simulink model "observe_2021a"  (R2021a)
settings: Solver=FixedStepAuto  StartTime=0.0  StopTime=15  RelTol=1e-3
model workspace (MAT data in the model file):
  A = 1
values from neighbouring files (symbols this model uses):
  Ap = [0, 1, 0; -C*df0*I0/mass, 0, -2*C*f0*I0/mass; 0, 0, -R/L]    [sliding_mode_control.m]    (also in system_state_feedback.m = [0, 1, 0; -C*df0*I0^2/mass, 0, -2*C*f0*I0/mass; 0, 0, -R/L]; system_state_feedback_observer.m = [0, 1, 0; -C*df0*I0^2/mass, 0, -2*C*f0*I0/mass; 0, 0, -R/L])
  Bp = [0; 0; 1/L]    [sliding_mode_control.m]    (also in system_state_feedback.m; system_state_feedback_observer.m)
  Cp = [1, 0, 0; 1, 0, 1]    [sliding_mode_control.m]    (also in system_state_feedback.m = [1, 0, 0; 0, 0, 1]; system_state_feedback_observer.m = [1, 0, 0; 0, 0, 1])
  D = [-C*df0*I0^2/mass-lambda^2, -2*C*f0*I0/mass]    [system_state_feedback_observer.m]
  I0 = sqrt((mass*grav)/(C*f_mag_y(y0)))    [sliding_mode_control.m]    (also in system_state_feedback.m = f_I0(y0); system_state_feedback_observer.m)
  K = place(Ap,Bp,p)    [sliding_mode_control.m]    (also in system_state_feedback.m; system_state_feedback_observer.m)
  L = 3.165    [feedback_linealization.m]    (also in sliding_mode_control.m; system_state_feedback.m; system_state_feedback_observer.m = place(Apt,Cpt,q))
  lambda = 200    [system_state_feedback_observer.m]
  V = [1,0;lambda,0;0,1]    [system_state_feedback_observer.m]
  V0 = R*I0    [sliding_mode_control.m]    (also in system_state_feedback.m = f_V0(y0); system_state_feedback_observer.m)
  W = [0;1;0]    [system_state_feedback_observer.m]
  y0 = 0.018    [sliding_mode_control.m]    (also in system_state_feedback.m = 0.03; system_state_feedback_observer.m = 0.02)
undefined symbols (not defined in the file or in its folder): National_Instruments, PCIe
libraries: sldrtlib x7
settings Model: SimulationMode=external  Creator=磁気浮上  LastModifiedBy=磁気浮上
settings SolverCC: AlgebraicLoopSolver=TrustRegion  DecoupledContinuousIntegration=on  MinimalZcImpactIntegration=on
settings DataIOCC: ReturnWorkspaceOutputs=off
settings DebuggingCC: SFMachineParentedDataDiag=warning  ArithmeticOperatorsInVariantConditions=warning
settings SFSimCC: SimUseLocalCustomCode=off  CustomCodeUndefinedFunction=UseInterfaceOnly
settings RTWCC: Description=Simulink Desktop Real-Time  SystemTargetFile=sldrt.tlc  TemplateMakefile=sldrt.tmf  RTWUseLocalCustomCode=off  RTWCompilerOptimization=on
settings CodeAppCC: MaxIdLength=95
settings SimulinkDesktopRealTimeCC: TargetPreCompLibLocation=C:\Program Files\MATLAB\R2021a\toolbox\sldrt\lib\win64

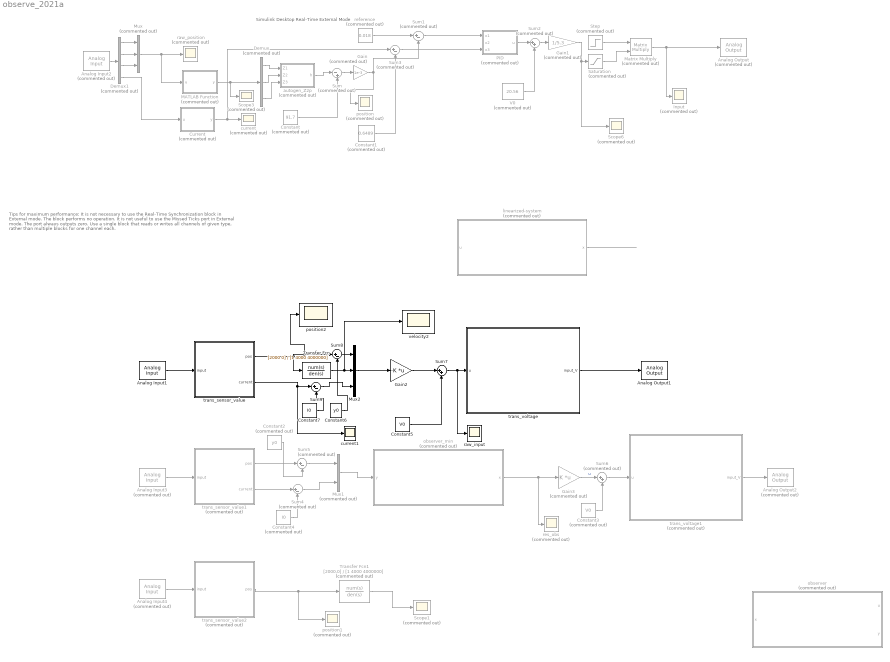
== system observe_2021a ==
  note: Simulink Desktop Real-Time External Mode
  note: Tips for maximum performance:
      |
      | It is not necessary to use the Real-Time Synchronization block in External mode. The block performs no operation.
      | It is not useful to use the Missed Ticks port in External mode. The port always outputs zero.
      | Use a single block that reads or writes all channels of given type, rather than multiple blocks for one channel each.
  Analog Input1 : sldrtlib/Analog Input  SampleTime=0.001  MaxMissedTicks=10  ShowMissedTicks=off  YieldWhenWaiting=off  DrvName=National_Instruments/PCIe-6361  DrvAddress=4294967295  DrvOptions=[0 0 0 0 0 0 0]  Channels=[1 2 3 5]  RangeMode=1  VoltRange=1  DataType=1
      settings: AttributesFormatString=National Instruments\nPCIe-6361 [auto]
  Analog Input2 : sldrtlib/Analog Input  Commented=on  SampleTime=0.001  MaxMissedTicks=10  ShowMissedTicks=off  YieldWhenWaiting=off  DrvName=National_Instruments/PCIe-6361  DrvAddress=4294967295  DrvOptions=[0 0 0 0 0 0 0]  Channels=[1 2 3 5]  RangeMode=1  VoltRange=1  DataType=1
      settings: AttributesFormatString=National Instruments\nPCIe-6361 [auto]
  Analog Input3 : sldrtlib/Analog Input  Commented=on  SampleTime=0.001  MaxMissedTicks=10  ShowMissedTicks=off  YieldWhenWaiting=off  DrvName=National_Instruments/PCIe-6361  DrvAddress=4294967295  DrvOptions=[0 0 0 0 0 0 0]  Channels=[1 2 3 5]  RangeMode=1  VoltRange=1  DataType=1
      settings: AttributesFormatString=National Instruments\nPCIe-6361 [auto]
  Analog Input4 : sldrtlib/Analog Input  Commented=on  SampleTime=0.0005  MaxMissedTicks=10  ShowMissedTicks=off  YieldWhenWaiting=off  DrvName=National_Instruments/PCIe-6361  DrvAddress=4294967295  DrvOptions=[0 0 0 0 0 0 0]  Channels=[1 2 3]  RangeMode=1  VoltRange=1  DataType=1
      settings: AttributesFormatString=National Instruments\nPCIe-6361 [auto]
  Analog Output : sldrtlib/Analog Output  Commented=on  SampleTime=0.001  MaxMissedTicks=10  ShowMissedTicks=off  YieldWhenWaiting=off  DrvName=National_Instruments/PCIe-6361  DrvAddress=4294967295  DrvOptions=[0 0 0 0 0 0 0]  Channels=1  RangeMode=1  VoltRange=1  InitialValue=[]  FinalValue=[]
      settings: AttributesFormatString=National Instruments\nPCIe-6361 [auto]
  Analog Output1 : sldrtlib/Analog Output  SampleTime=0.001  MaxMissedTicks=10  ShowMissedTicks=off  YieldWhenWaiting=off  DrvName=National_Instruments/PCIe-6361  DrvAddress=4294967295  DrvOptions=[0 0 0 0 0 0 0]  Channels=1  RangeMode=1  VoltRange=1  InitialValue=[]  FinalValue=[]
      settings: AttributesFormatString=National Instruments\nPCIe-6361 [auto]
  Analog Output2 : sldrtlib/Analog Output  Commented=on  SampleTime=0.001  MaxMissedTicks=10  ShowMissedTicks=off  YieldWhenWaiting=off  DrvName=National_Instruments/PCIe-6361  DrvAddress=4294967295  DrvOptions=[0 0 0 0 0 0 0]  Channels=1  RangeMode=1  VoltRange=1  InitialValue=[]  FinalValue=[]
      settings: AttributesFormatString=National Instruments\nPCIe-6361 [auto]
  Constant : Constant  Commented=on  Value=91.7
  Constant1 : Constant  Commented=on  Value=0.6489
  Constant2 : Constant  Commented=on  Value=y0
  Constant3 : Constant  Commented=on  Value=V0
  Constant4 : Constant  Commented=on  Value=I0
  Constant5 : Constant  Value=V0
  Constant6 : Constant  Value=y0
  Constant7 : Constant  Value=I0
  Current : MATLAB Function  Commented=on  TreatAsAtomicUnit=on
  Demux : Demux  Commented=on  Outputs=3
  Demux1 : Demux  Commented=on
  Gain : Gain  Commented=on  Gain=1e-3
  Gain1 : Gain  Commented=on  Gain=1/5.3
  Gain2 : Gain  Gain=-K  Multiplication=Matrix(K*u)
  Gain3 : Gain  Commented=on  Gain=K  Multiplication=Matrix(K*u)
  Input : Scope  Commented=on
  MATLAB Function : MATLAB Function  Commented=on  TreatAsAtomicUnit=on
  Matrix Multiply : Product  Commented=on  Multiplication=Matrix(*)
  Mux : Mux  Commented=on  Inputs=3
  Mux1 : Mux  Commented=on  Inputs=2
  Mux2 : Mux  Inputs=3
  PID : MATLAB Function  Commented=on  TreatAsAtomicUnit=on
  Saturation : Saturate  Commented=on  UpperLimit=10  LowerLimit=-10
  Scope1 : Scope  Commented=on
  Scope3 : Scope  Commented=on
  Scope6 : Scope  Commented=on
  Step : Step  Commented=on  Time=15  Before=1  After=0  SampleTime=0
  Sum : Sum  Commented=on  Inputs=|-+
  Sum{1,3..5} (4 alike) : Sum  Commented=on  Inputs=|+-
  Sum2 : Sum  Commented=on  Inputs=|++
  Sum6 : Sum  Commented=on  Inputs=|++
  Sum7 : Sum  Inputs=|++
  Sum8 : Sum  Inputs=|+-
  Sum9 : Sum  Inputs=|+-
  Transfer Fcn : TransferFcn  Numerator=[2000 0]  Denominator=[1 4000 4000000]
  Transfer Fcn1 : TransferFcn  Commented=on  Numerator=[2000,0]  Denominator=[1 4000 4000000]
  V0 : Constant  Commented=on  Value=20.56
  autogen_Z2p : MATLAB Function  Commented=on  TreatAsAtomicUnit=on
  current : Scope  Commented=on
  current1 : Scope
  linearized-system : Subsystem  Commented=on
  observer : Subsystem  Commented=on
  observer_min : Subsystem  Commented=on
  position : Scope  Commented=on
  position1 : Scope  Commented=on
  position2 : Scope
  raw_input : Scope
  raw_position : Scope  Commented=on
  reference : Constant  Commented=on  Value=0.018
  res_obs : Scope  Commented=on
  trans_sensor_value : Subsystem
  trans_sensor_value1 : Subsystem  Commented=on
  trans_sensor_value2 : Subsystem  Commented=on
  trans_voltage : Subsystem
  trans_voltage1 : Subsystem  Commented=on
  velocity2 : Scope
  wires:
  Step/1 -> Matrix Multiply/1
  Constant/1 -> Sum/2
  autogen_Z2p/1(h) -> Sum/1
  Matrix Multiply/1 -> Analog Output/1, Input/1
  MATLAB Function/1(y) -> Scope3/1, Demux/1
  Sum/1 -> Gain/1
  Demux/2 -> autogen_Z2p/2(Z2)
  Demux/1 -> autogen_Z2p/1(Z1)
  Saturation/1 -> Matrix Multiply/2
  Demux/3 -> autogen_Z2p/3(Z3)
  Current/1(y) -> Sum3/1, current/1
  Analog Input2/1 -> Demux1/1
  Demux1/1 -> Mux/1
  Demux1/4 -> Current/1(u)
  Demux1/3 -> Mux/3
  Demux1/2 -> Mux/2
  Mux/1 -> MATLAB Function/1(u), raw_position/1
  Gain/1 -> Sum1/2, position/1
  reference/1 -> Sum1/1
  Sum1/1 -> PID/1(x1)
  V0/1 -> Sum2/2
  PID/1(u) -> Sum2/1
  Sum2/1 -> Gain1/1
  Gain1/1 -> Saturation/1, Scope6/1
  Sum3/1 -> PID/3(x3)
  Constant1/1 -> Sum3/2
  linearized-system/1(x) -> ?
  Analog Input1/1 -> trans_sensor_value/1(input)
  trans_sensor_value/1(pos) -> position2/1, Sum8/1, Transfer Fcn/1
  trans_sensor_value/2(current) -> Sum9/1, current1/1
  Gain2/1 -> Sum7/1
  trans_voltage/1(input_V) -> Analog Output1/1
  trans_voltage1/1(input_V) -> Analog Output2/1
  trans_sensor_value1/1(pos) -> Sum5/1
  Analog Input3/1 -> trans_sensor_value1/1(input)
  Gain3/1 -> Sum6/1  "u"
  Transfer Fcn/1 -> velocity2/1, Mux2/2
  Mux2/1 -> Gain2/1
  Mux1/1 -> observer_min/1(y)
  observer_min/1(x) -> res_obs/1, Gain3/1
  Constant4/1 -> Sum4/2
  trans_sensor_value1/2(current) -> Sum4/1
  Sum4/1 -> Mux1/2
  Constant2/1 -> Sum5/2
  Sum5/1 -> Mux1/1
  Constant3/1 -> Sum6/2
  Sum6/1 -> trans_voltage1/1(u)
  trans_sensor_value2/1(pos) -> position1/1, Transfer Fcn1/1
  Transfer Fcn1/1 -> Scope1/1
  Analog Input4/1 -> trans_sensor_value2/1(input)
  Constant5/1 -> Sum7/2
  Sum7/1 -> raw_input/1, trans_voltage/1(u)
  Constant6/1 -> Sum8/2
  Sum8/1 -> Mux2/1
  Constant7/1 -> Sum9/2
  Sum9/1 -> Mux2/3

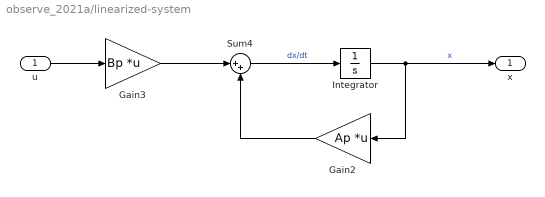
== system observe_2021a/linearized-system ==
  u : Inport
  Gain2 : Gain  Gain=Ap  Multiplication=Matrix(K*u)
  Gain3 : Gain  Gain=Bp  Multiplication=Matrix(K*u)
  Integrator : Integrator
  Sum4 : Sum  Inputs=|++
  x : Outport
  wires:
  Gain3/1 -> Sum4/1
  Gain2/1 -> Sum4/2
  u/1 -> Gain3/1
  Integrator/1 -> Gain2/1, x/1  "x"
  Sum4/1 -> Integrator/1  "dx/dt"

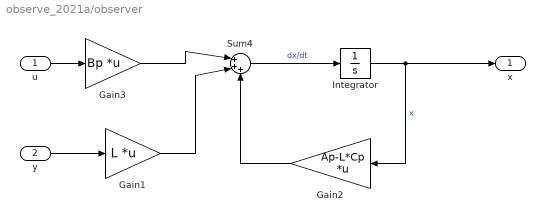
== system observe_2021a/observer ==
  u : Inport
  y : Inport  Port=2
  Gain1 : Gain  Gain=L  Multiplication=Matrix(K*u)
  Gain2 : Gain  Gain=Ap-L*Cp  Multiplication=Matrix(K*u)
  Gain3 : Gain  Gain=Bp  Multiplication=Matrix(K*u)
  Integrator : Integrator
  Sum4 : Sum  Inputs=|+++
  x : Outport
  wires:
  Gain3/1 -> Sum4/1
  Gain2/1 -> Sum4/3
  Integrator/1 -> Gain2/1, x/1  "x"
  Sum4/1 -> Integrator/1  "dx/dt"
  y/1 -> Gain1/1
  Gain1/1 -> Sum4/2
  u/1 -> Gain3/1

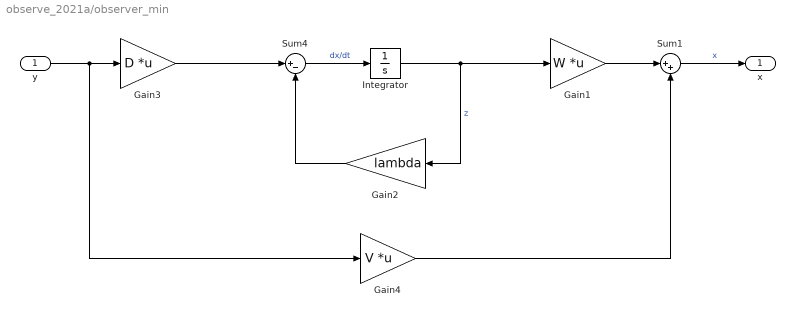
== system observe_2021a/observer_min ==
  y : Inport
  Gain1 : Gain  Gain=W  Multiplication=Matrix(K*u)
  Gain2 : Gain  Gain=lambda
  Gain3 : Gain  Gain=D  Multiplication=Matrix(K*u)
  Gain4 : Gain  Gain=V  Multiplication=Matrix(K*u)
  Integrator : Integrator
  Sum1 : Sum  Inputs=|++
  Sum4 : Sum  Inputs=|+-
  x : Outport
  wires:
  Gain2/1 -> Sum4/2
  Integrator/1 -> Gain1/1, Gain2/1  "z"
  Sum4/1 -> Integrator/1  "dx/dt"
  y/1 -> Gain4/1, Gain3/1
  Gain3/1 -> Sum4/1
  Gain1/1 -> Sum1/1
  Gain4/1 -> Sum1/2
  Sum1/1 -> x/1  "x"

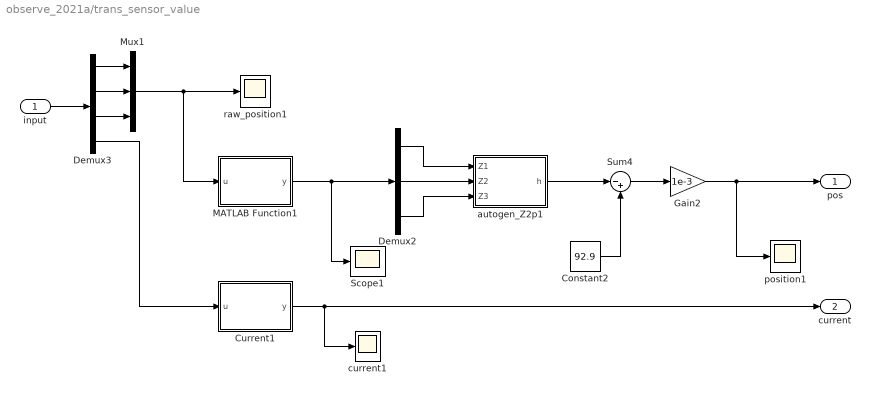
== system observe_2021a/trans_sensor_value ==
  input : Inport
  Constant2 : Constant  Value=92.9
  Current1 : MATLAB Function  TreatAsAtomicUnit=on
  Demux2 : Demux  Outputs=3
  Demux3 : Demux
  Gain2 : Gain  Gain=1e-3
  MATLAB Function1 : MATLAB Function  TreatAsAtomicUnit=on
  Mux1 : Mux  Inputs=3
  Scope1 : Scope
  Sum4 : Sum  Inputs=|-+
  autogen_Z2p1 : MATLAB Function  TreatAsAtomicUnit=on
  current1 : Scope
  position1 : Scope
  raw_position1 : Scope
  pos : Outport
  current : Outport  Port=2
  wires:
  Gain2/1 -> pos/1, position1/1
  MATLAB Function1/1(y) -> Demux2/1, Scope1/1
  Mux1/1 -> MATLAB Function1/1(u), raw_position1/1
  Sum4/1 -> Gain2/1
  Demux3/1 -> Mux1/1
  Demux2/1 -> autogen_Z2p1/1(Z1)
  autogen_Z2p1/1(h) -> Sum4/1
  Demux3/3 -> Mux1/3
  Demux2/3 -> autogen_Z2p1/3(Z3)
  Demux2/2 -> autogen_Z2p1/2(Z2)
  Demux3/4 -> Current1/1(u)
  Demux3/2 -> Mux1/2
  Current1/1(y) -> current/1, current1/1
  Constant2/1 -> Sum4/2
  input/1 -> Demux3/1

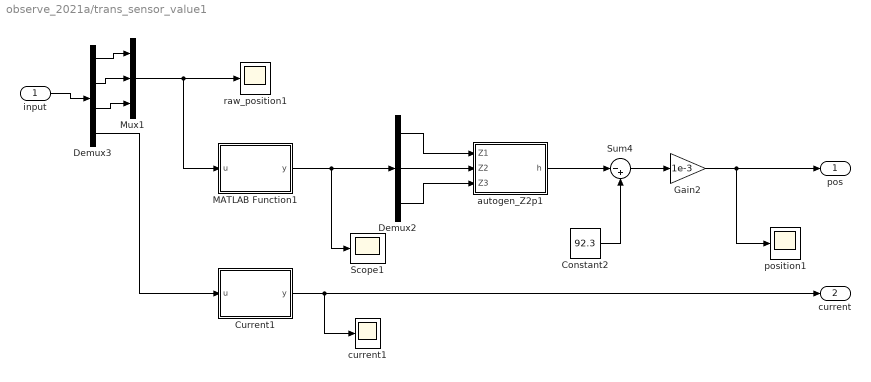
== system observe_2021a/trans_sensor_value1 ==
  input : Inport
  Constant2 : Constant  Value=92.3
  Current1 : MATLAB Function  TreatAsAtomicUnit=on
  Demux2 : Demux  Outputs=3
  Demux3 : Demux
  Gain2 : Gain  Gain=1e-3
  MATLAB Function1 : MATLAB Function  TreatAsAtomicUnit=on
  Mux1 : Mux  Inputs=3
  Scope1 : Scope
  Sum4 : Sum  Inputs=|-+
  autogen_Z2p1 : MATLAB Function  TreatAsAtomicUnit=on
  current1 : Scope
  position1 : Scope
  raw_position1 : Scope
  pos : Outport
  current : Outport  Port=2
  wires:
  Gain2/1 -> pos/1, position1/1
  MATLAB Function1/1(y) -> Demux2/1, Scope1/1
  Mux1/1 -> MATLAB Function1/1(u), raw_position1/1
  Sum4/1 -> Gain2/1
  Demux3/1 -> Mux1/1
  Demux2/1 -> autogen_Z2p1/1(Z1)
  autogen_Z2p1/1(h) -> Sum4/1
  Demux3/3 -> Mux1/3
  Demux2/3 -> autogen_Z2p1/3(Z3)
  Demux2/2 -> autogen_Z2p1/2(Z2)
  Demux3/4 -> Current1/1(u)
  Demux3/2 -> Mux1/2
  Current1/1(y) -> current/1, current1/1
  Constant2/1 -> Sum4/2
  input/1 -> Demux3/1

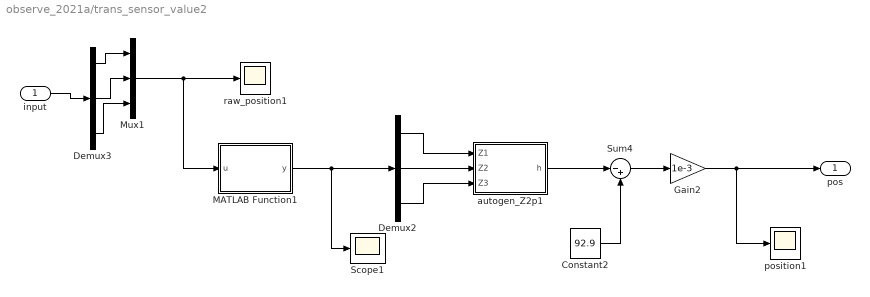
== system observe_2021a/trans_sensor_value2 ==
  input : Inport
  Constant2 : Constant  Value=92.9
  Demux2 : Demux  Outputs=3
  Demux3 : Demux  Outputs=3
  Gain2 : Gain  Gain=1e-3
  MATLAB Function1 : MATLAB Function  TreatAsAtomicUnit=on
  Mux1 : Mux  Inputs=3
  Scope1 : Scope
  Sum4 : Sum  Inputs=|-+
  autogen_Z2p1 : MATLAB Function  TreatAsAtomicUnit=on
  position1 : Scope
  raw_position1 : Scope
  pos : Outport
  wires:
  Gain2/1 -> pos/1, position1/1
  MATLAB Function1/1(y) -> Demux2/1, Scope1/1
  Mux1/1 -> MATLAB Function1/1(u), raw_position1/1
  Sum4/1 -> Gain2/1
  Demux3/1 -> Mux1/1
  Demux2/1 -> autogen_Z2p1/1(Z1)
  autogen_Z2p1/1(h) -> Sum4/1
  Demux3/3 -> Mux1/3
  Demux2/3 -> autogen_Z2p1/3(Z3)
  Demux2/2 -> autogen_Z2p1/2(Z2)
  Demux3/2 -> Mux1/2
  Constant2/1 -> Sum4/2
  input/1 -> Demux3/1

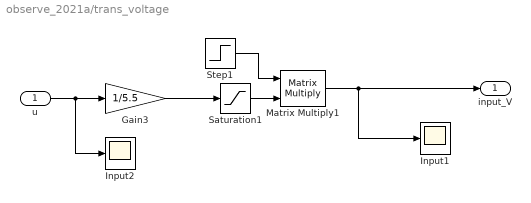
== system observe_2021a/trans_voltage ==
  u : Inport
  Gain3 : Gain  Gain=1/5.5
  Input1 : Scope
  Input2 : Scope
  Matrix Multiply1 : Product  Multiplication=Matrix(*)
  Saturation1 : Saturate  UpperLimit=10  LowerLimit=-10
  Step1 : Step  Time=10  Before=1  After=0  SampleTime=0
  input_V : Outport
  wires:
  Gain3/1 -> Saturation1/1
  Step1/1 -> Matrix Multiply1/1
  Matrix Multiply1/1 -> input_V/1, Input1/1
  u/1 -> Input2/1, Gain3/1
  Saturation1/1 -> Matrix Multiply1/2

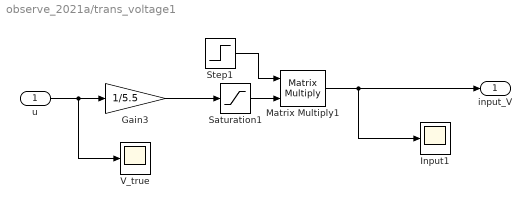
== system observe_2021a/trans_voltage1 ==
  u : Inport
  Gain3 : Gain  Gain=1/5.5
  Input1 : Scope
  Matrix Multiply1 : Product  Multiplication=Matrix(*)
  Saturation1 : Saturate  UpperLimit=10  LowerLimit=-10
  Step1 : Step  Time=15  Before=1  After=0  SampleTime=0
  V_true : Scope
  input_V : Outport
  wires:
  Gain3/1 -> Saturation1/1
  Step1/1 -> Matrix Multiply1/1
  Matrix Multiply1/1 -> input_V/1, Input1/1
  Saturation1/1 -> Matrix Multiply1/2
  u/1 -> V_true/1, Gain3/1

== matlab function observe_2021a/autogen_Z2p ==
  data: Z1 input; h output; Z2 input; Z3 input
function h = autogen_Z2p(Z1,Z2,Z3)
%#codegen

%    This function was generated by the Symbolic Math Toolbox version 8.7.
%    09-Feb-2022 18:15:15

t2 = Z1.^2;
t3 = Z1.^3;
t4 = Z2.^2;
t5 = Z2.^3;
t6 = Z3.^2;
t7 = Z3.^3;
t8 = Z1.*3.21e+2;
t9 = Z2.*1.297e+3;
t10 = Z3.*1.763e+3;
t11 = Z3.*2.576e+3;
t12 = Z2.*2.897e+3;
t13 = Z1.*3.06e+3;
t24 = Z2.*Z3.*1.0352122e+11;
t25 = Z2.*Z3.*2.0704244e+11;
t26 = Z1.*Z3.*9.135768e+10;
t27 = Z1.*Z3.*1.8271536e+11;
t28 = Z1.*Z2.*1.9595028e+11;
t29 = Z1.*Z2.*9.797514e+10;
t39 = Z1.*4.8999911281101e+13;
t41 = Z3.*4.7733218776365e+13;
t48 = Z2.*4.6020599945112e+13;
t56 = Z1.*Z3.*2.511664935e+13;
t57 = Z1.*1.42753730002578e+14;
t58 = Z2.*Z3.*5.124007469e+13;
t68 = Z1.*Z2.*4.264372839e+13;
t80 = Z1.*Z2.*1.7692425141e+14;
t82 = Z1.*Z3.*1.4293441815e+14;
t88 = Z2.*Z3.*2.2089361633e+14;
t14 = -t12;
t15 = -t13;
t16 = t2.*3.21e+6;
t17 = t4.*1.297e+7;
t18 = t6.*1.763e+7;
t19 = t6.*2.576e+7;
t20 = t4.*2.897e+7;
t21 = t2.*3.06e+7;
t30 = t4.*2.0149636e+11;
t31 = Z1.*t6.*4.567884e+10;
t32 = Z3.*t2.*4.567884e+10;
t33 = t2.*9.466641e+10;
t34 = t3.*9.466641e+10;
t35 = -t24;
t36 = t2.*1.8933282e+11;
t37 = -t25;
t38 = -t26;
t40 = t6.*1.948789e+11;
t42 = Z2.*t6.*5.176061e+10;
t43 = Z3.*t4.*5.176061e+10;
t44 = t4.*1.0074818e+11;
t45 = t5.*1.0074818e+11;
t46 = -t27;
t47 = -t28;
t49 = t6.*9.743945e+10;
t50 = t7.*9.743945e+10;
t51 = Z1.*t4.*4.898757e+10;
t52 = Z2.*t2.*4.898757e+10;
t53 = -t29;
t54 = Z2.*t3.*3.21e+10;
t55 = Z3.*t3.*3.21e+10;
t59 = Z1.*t7.*2.576e+11;
t60 = Z2.*t7.*2.576e+11;
t61 = Z1.*t7.*1.763e+11;
t62 = Z2.*t7.*1.763e+11;
t63 = Z1.*t5.*1.297e+11;
t64 = Z3.*t5.*1.297e+11;
t65 = Z2.*Z3.*t2.*4.66e+10;
t66 = Z2.*t3.*3.06e+11;
t67 = Z3.*t3.*3.06e+11;
t69 = Z1.*t5.*2.897e+11;
t70 = Z3.*t5.*2.897e+11;
t72 = t2.*1.699491663e+13;
t73 = Z1.*Z3.*t4.*4.823e+11;
t74 = Z2.*Z3.*t2.*5.473e+11;
t75 = Z1.*Z2.*t6.*4.357e+11;
t76 = Z1.*Z3.*t4.*2.255e+11;
t77 = -t58;
t79 = t2.*3.388018887e+13;
t84 = t4.*t6.*4.66e+10;
t86 = t6.*4.584717173e+13;
t87 = Z1.*Z2.*t6.*3.218e+11;
t91 = t4.*8.912494397e+13;
t92 = t2.*t6.*4.823e+11;
t93 = t4.*t6.*5.473e+11;
t94 = t2.*t4.*4.357e+11;
t96 = t2.*t6.*2.255e+11;
t98 = -t80;
t99 = t6.*9.788848349e+13;
t103 = t2.*t4.*3.218e+11;
t104 = -t88;
t105 = t4.*1.1408216305e+14;
t110 = t2.*2.85507460005156e+18;
t22 = -t20;
t23 = -t21;
t71 = -t55;
t78 = -t60;
t81 = -t62;
t83 = -t63;
t85 = -t66;
t89 = -t70;
t90 = -t73;
t95 = -t76;
t97 = -t79;
t100 = t8+t11+t14;
t101 = -t86;
t102 = -t87;
t106 = -t92;
t107 = -t96;
t108 = t9+t10+t15;
t109 = -t103;
t117 = t30+t36+t37+t40+t46+t47+1.42753730002578e+14;
t118 = t33+t35+t38+t44+t49+t53+7.1376865001289e+13;
t111 = t16+t19+t22-2.275477497e+9;
t112 = t17+t18+t23+3.0399800799e+10;
t119 = 1.0./t118;
t120 = 1.0./t117;
t113 = t111.^2;
t114 = t112.^2;
t115 = t100.*t111;
t116 = t108.*t112;
t121 = t110+t113+t114-2.569567140046404e+21;
t122 = t57+t115+t116;
t123 = t122.^2;
t125 = t118.*t121;
t124 = t123.*1.0e+4;
t126 = -t125;
t127 = t124+t126;
t128 = sqrt(t127);
t129 = t128./1.0e+2;
t130 = Z1.*t128.*3.799498679230342e-3;
t131 = Z1.*t128.*3.621952011976588e-2;
t132 = Z2.*t128.*1.535186849520796e-2;
t133 = Z3.*t128.*2.086765162455792e-2;
t134 = Z3.*t128.*3.049068098971141e-2;
t135 = Z2.*t128.*3.429017966894175e-2;
mt1 = [(t119.*(t61+t64+t65+t67+t72+t75+t77+t81+t82+t83+t84+t85+t90+t94+t98+t101+t105+t106+t130+t134-t135+1.922433295028705e+16))./2.0e+2,(t119.*(t61+t64+t65+t67+t72+t75+t77+t81+t82+t83+t84+t85+t90+t94+t98+t101+t105+t106-t130-t134+t135+1.922433295028705e+16))./2.0e+2,(t119.*(t54-t55+t56+t59-t60+t68+t69+t74+t89+t91+t93+t95+t97+t99+t102+t104+t107+t109+t131-t132-t133+3.556391874974202e+16))./2.0e+2];
mt2 = [(t119.*(t54+t56+t59+t68+t69+t71+t74+t78+t89+t91+t93+t95+t97+t99+t102+t104+t107+t109-t131+t132+t133+3.556391874974202e+16))./2.0e+2,t120.*(-t31-t32+t34+t39+t41-t42-t43+t45+t48+t50-t51-t52+t129)+3.0e+1,-t120.*(t31+t32-t34-t39-t41+t42+t43-t45-t48-t50+t51+t52+t129)+3.0e+1];
pv = reshape([mt1,mt2],2,3);

if pv(1,3)>0
    h=pv(1,3);
else
    h=pv(2,3);
end

== matlab function observe_2021a/trans_sensor_value/Current1 ==
  data: u input; y output
function y = fcn(u)
%u:バイポーラ電源の出力値（V）（電流を観測）、y:バイポーラ電源が流している電流(A)
    %出力電圧値が距離に変換されます。
    y=(3.01/6.23)*u;

== matlab function observe_2021a/Current ==
  data: u input; y output
function y = fcn(u)
%u:バイポーラ電源の出力値（V）（電流を観測）、y:バイポーラ電源が流している電流(A)
    %出力電圧値が距離に変換されます。
    y=(3.01/6.23)*u;

== matlab function observe_2021a/PID ==
  data: x1 input; u output; x2 input; x3 input
function u = autogen_Z2p(x1,x2,x3)
%#codegen

%    This function was generated by the Symbolic Math Toolbox version 8.7.
%    18-Apr-2022 15:37:02



K = [ -1545, -133, 6.3];
x = [x1; x2; x3];

u = -K*x;

== matlab function observe_2021a/trans_sensor_value/MATLAB Function1 ==
  data: u input; y output
function y = fcn(u)
%u:光学センサの出力(V)、y:光学センサの出力PV値(mm)
    %出力スケーリングを行っています(フリーレンジ)。（光学センサの設定10,P.4-27）
    %PV値範囲を0～-50、出力電圧範囲を-5～5としているので、以下の式に従って
    %電圧値が距離に変換されます。
    y=(u-5*ones(3,1))*(-5);
% y = u;

== matlab function observe_2021a/trans_sensor_value/autogen_Z2p1 ==
  data: Z1 input; h output; Z2 input; Z3 input
function h = autogen_Z2p(Z1,Z2,Z3)
%#codegen

%    This function was generated by the Symbolic Math Toolbox version 8.7.
%    09-Feb-2022 18:15:15

t2 = Z1.^2;
t3 = Z1.^3;
t4 = Z2.^2;
t5 = Z2.^3;
t6 = Z3.^2;
t7 = Z3.^3;
t8 = Z1.*3.21e+2;
t9 = Z2.*1.297e+3;
t10 = Z3.*1.763e+3;
t11 = Z3.*2.576e+3;
t12 = Z2.*2.897e+3;
t13 = Z1.*3.06e+3;
t24 = Z2.*Z3.*1.0352122e+11;
t25 = Z2.*Z3.*2.0704244e+11;
t26 = Z1.*Z3.*9.135768e+10;
t27 = Z1.*Z3.*1.8271536e+11;
t28 = Z1.*Z2.*1.9595028e+11;
t29 = Z1.*Z2.*9.797514e+10;
t39 = Z1.*4.8999911281101e+13;
t41 = Z3.*4.7733218776365e+13;
t48 = Z2.*4.6020599945112e+13;
t56 = Z1.*Z3.*2.511664935e+13;
t57 = Z1.*1.42753730002578e+14;
t58 = Z2.*Z3.*5.124007469e+13;
t68 = Z1.*Z2.*4.264372839e+13;
t80 = Z1.*Z2.*1.7692425141e+14;
t82 = Z1.*Z3.*1.4293441815e+14;
t88 = Z2.*Z3.*2.2089361633e+14;
t14 = -t12;
t15 = -t13;
t16 = t2.*3.21e+6;
t17 = t4.*1.297e+7;
t18 = t6.*1.763e+7;
t19 = t6.*2.576e+7;
t20 = t4.*2.897e+7;
t21 = t2.*3.06e+7;
t30 = t4.*2.0149636e+11;
t31 = Z1.*t6.*4.567884e+10;
t32 = Z3.*t2.*4.567884e+10;
t33 = t2.*9.466641e+10;
t34 = t3.*9.466641e+10;
t35 = -t24;
t36 = t2.*1.8933282e+11;
t37 = -t25;
t38 = -t26;
t40 = t6.*1.948789e+11;
t42 = Z2.*t6.*5.176061e+10;
t43 = Z3.*t4.*5.176061e+10;
t44 = t4.*1.0074818e+11;
t45 = t5.*1.0074818e+11;
t46 = -t27;
t47 = -t28;
t49 = t6.*9.743945e+10;
t50 = t7.*9.743945e+10;
t51 = Z1.*t4.*4.898757e+10;
t52 = Z2.*t2.*4.898757e+10;
t53 = -t29;
t54 = Z2.*t3.*3.21e+10;
t55 = Z3.*t3.*3.21e+10;
t59 = Z1.*t7.*2.576e+11;
t60 = Z2.*t7.*2.576e+11;
t61 = Z1.*t7.*1.763e+11;
t62 = Z2.*t7.*1.763e+11;
t63 = Z1.*t5.*1.297e+11;
t64 = Z3.*t5.*1.297e+11;
t65 = Z2.*Z3.*t2.*4.66e+10;
t66 = Z2.*t3.*3.06e+11;
t67 = Z3.*t3.*3.06e+11;
t69 = Z1.*t5.*2.897e+11;
t70 = Z3.*t5.*2.897e+11;
t72 = t2.*1.699491663e+13;
t73 = Z1.*Z3.*t4.*4.823e+11;
t74 = Z2.*Z3.*t2.*5.473e+11;
t75 = Z1.*Z2.*t6.*4.357e+11;
t76 = Z1.*Z3.*t4.*2.255e+11;
t77 = -t58;
t79 = t2.*3.388018887e+13;
t84 = t4.*t6.*4.66e+10;
t86 = t6.*4.584717173e+13;
t87 = Z1.*Z2.*t6.*3.218e+11;
t91 = t4.*8.912494397e+13;
t92 = t2.*t6.*4.823e+11;
t93 = t4.*t6.*5.473e+11;
t94 = t2.*t4.*4.357e+11;
t96 = t2.*t6.*2.255e+11;
t98 = -t80;
t99 = t6.*9.788848349e+13;
t103 = t2.*t4.*3.218e+11;
t104 = -t88;
t105 = t4.*1.1408216305e+14;
t110 = t2.*2.85507460005156e+18;
t22 = -t20;
t23 = -t21;
t71 = -t55;
t78 = -t60;
t81 = -t62;
t83 = -t63;
t85 = -t66;
t89 = -t70;
t90 = -t73;
t95 = -t76;
t97 = -t79;
t100 = t8+t11+t14;
t101 = -t86;
t102 = -t87;
t106 = -t92;
t107 = -t96;
t108 = t9+t10+t15;
t109 = -t103;
t117 = t30+t36+t37+t40+t46+t47+1.42753730002578e+14;
t118 = t33+t35+t38+t44+t49+t53+7.1376865001289e+13;
t111 = t16+t19+t22-2.275477497e+9;
t112 = t17+t18+t23+3.0399800799e+10;
t119 = 1.0./t118;
t120 = 1.0./t117;
t113 = t111.^2;
t114 = t112.^2;
t115 = t100.*t111;
t116 = t108.*t112;
t121 = t110+t113+t114-2.569567140046404e+21;
t122 = t57+t115+t116;
t123 = t122.^2;
t125 = t118.*t121;
t124 = t123.*1.0e+4;
t126 = -t125;
t127 = t124+t126;
t128 = sqrt(t127);
t129 = t128./1.0e+2;
t130 = Z1.*t128.*3.799498679230342e-3;
t131 = Z1.*t128.*3.621952011976588e-2;
t132 = Z2.*t128.*1.535186849520796e-2;
t133 = Z3.*t128.*2.086765162455792e-2;
t134 = Z3.*t128.*3.049068098971141e-2;
t135 = Z2.*t128.*3.429017966894175e-2;
mt1 = [(t119.*(t61+t64+t65+t67+t72+t75+t77+t81+t82+t83+t84+t85+t90+t94+t98+t101+t105+t106+t130+t134-t135+1.922433295028705e+16))./2.0e+2,(t119.*(t61+t64+t65+t67+t72+t75+t77+t81+t82+t83+t84+t85+t90+t94+t98+t101+t105+t106-t130-t134+t135+1.922433295028705e+16))./2.0e+2,(t119.*(t54-t55+t56+t59-t60+t68+t69+t74+t89+t91+t93+t95+t97+t99+t102+t104+t107+t109+t131-t132-t133+3.556391874974202e+16))./2.0e+2];
mt2 = [(t119.*(t54+t56+t59+t68+t69+t71+t74+t78+t89+t91+t93+t95+t97+t99+t102+t104+t107+t109-t131+t132+t133+3.556391874974202e+16))./2.0e+2,t120.*(-t31-t32+t34+t39+t41-t42-t43+t45+t48+t50-t51-t52+t129)+3.0e+1,-t120.*(t31+t32-t34-t39-t41+t42+t43-t45-t48-t50+t51+t52+t129)+3.0e+1];
pv = reshape([mt1,mt2],2,3);

if pv(1,3)>0
    h=pv(1,3);
else
    h=pv(2,3);
end

== matlab function observe_2021a/trans_sensor_value1/Current1 ==
  data: u input; y output
function y = fcn(u)
%u:バイポーラ電源の出力値（V）（電流を観測）、y:バイポーラ電源が流している電流(A)
    %出力電圧値が距離に変換されます。
    y=(3.01/6.23)*u;

== matlab function observe_2021a/trans_sensor_value1/MATLAB Function1 ==
  data: u input; y output
function y = fcn(u)
%u:光学センサの出力(V)、y:光学センサの出力PV値(mm)
    %出力スケーリングを行っています(フリーレンジ)。（光学センサの設定10,P.4-27）
    %PV値範囲を0～-50、出力電圧範囲を-5～5としているので、以下の式に従って
    %電圧値が距離に変換されます。
    y=(u-5*ones(3,1))*(-5);
% y = u;

== matlab function observe_2021a/trans_sensor_value1/autogen_Z2p1 ==
  data: Z1 input; h output; Z2 input; Z3 input
function h = autogen_Z2p(Z1,Z2,Z3)
%#codegen

%    This function was generated by the Symbolic Math Toolbox version 8.7.
%    09-Feb-2022 18:15:15

t2 = Z1.^2;
t3 = Z1.^3;
t4 = Z2.^2;
t5 = Z2.^3;
t6 = Z3.^2;
t7 = Z3.^3;
t8 = Z1.*3.21e+2;
t9 = Z2.*1.297e+3;
t10 = Z3.*1.763e+3;
t11 = Z3.*2.576e+3;
t12 = Z2.*2.897e+3;
t13 = Z1.*3.06e+3;
t24 = Z2.*Z3.*1.0352122e+11;
t25 = Z2.*Z3.*2.0704244e+11;
t26 = Z1.*Z3.*9.135768e+10;
t27 = Z1.*Z3.*1.8271536e+11;
t28 = Z1.*Z2.*1.9595028e+11;
t29 = Z1.*Z2.*9.797514e+10;
t39 = Z1.*4.8999911281101e+13;
t41 = Z3.*4.7733218776365e+13;
t48 = Z2.*4.6020599945112e+13;
t56 = Z1.*Z3.*2.511664935e+13;
t57 = Z1.*1.42753730002578e+14;
t58 = Z2.*Z3.*5.124007469e+13;
t68 = Z1.*Z2.*4.264372839e+13;
t80 = Z1.*Z2.*1.7692425141e+14;
t82 = Z1.*Z3.*1.4293441815e+14;
t88 = Z2.*Z3.*2.2089361633e+14;
t14 = -t12;
t15 = -t13;
t16 = t2.*3.21e+6;
t17 = t4.*1.297e+7;
t18 = t6.*1.763e+7;
t19 = t6.*2.576e+7;
t20 = t4.*2.897e+7;
t21 = t2.*3.06e+7;
t30 = t4.*2.0149636e+11;
t31 = Z1.*t6.*4.567884e+10;
t32 = Z3.*t2.*4.567884e+10;
t33 = t2.*9.466641e+10;
t34 = t3.*9.466641e+10;
t35 = -t24;
t36 = t2.*1.8933282e+11;
t37 = -t25;
t38 = -t26;
t40 = t6.*1.948789e+11;
t42 = Z2.*t6.*5.176061e+10;
t43 = Z3.*t4.*5.176061e+10;
t44 = t4.*1.0074818e+11;
t45 = t5.*1.0074818e+11;
t46 = -t27;
t47 = -t28;
t49 = t6.*9.743945e+10;
t50 = t7.*9.743945e+10;
t51 = Z1.*t4.*4.898757e+10;
t52 = Z2.*t2.*4.898757e+10;
t53 = -t29;
t54 = Z2.*t3.*3.21e+10;
t55 = Z3.*t3.*3.21e+10;
t59 = Z1.*t7.*2.576e+11;
t60 = Z2.*t7.*2.576e+11;
t61 = Z1.*t7.*1.763e+11;
t62 = Z2.*t7.*1.763e+11;
t63 = Z1.*t5.*1.297e+11;
t64 = Z3.*t5.*1.297e+11;
t65 = Z2.*Z3.*t2.*4.66e+10;
t66 = Z2.*t3.*3.06e+11;
t67 = Z3.*t3.*3.06e+11;
t69 = Z1.*t5.*2.897e+11;
t70 = Z3.*t5.*2.897e+11;
t72 = t2.*1.699491663e+13;
t73 = Z1.*Z3.*t4.*4.823e+11;
t74 = Z2.*Z3.*t2.*5.473e+11;
t75 = Z1.*Z2.*t6.*4.357e+11;
t76 = Z1.*Z3.*t4.*2.255e+11;
t77 = -t58;
t79 = t2.*3.388018887e+13;
t84 = t4.*t6.*4.66e+10;
t86 = t6.*4.584717173e+13;
t87 = Z1.*Z2.*t6.*3.218e+11;
t91 = t4.*8.912494397e+13;
t92 = t2.*t6.*4.823e+11;
t93 = t4.*t6.*5.473e+11;
t94 = t2.*t4.*4.357e+11;
t96 = t2.*t6.*2.255e+11;
t98 = -t80;
t99 = t6.*9.788848349e+13;
t103 = t2.*t4.*3.218e+11;
t104 = -t88;
t105 = t4.*1.1408216305e+14;
t110 = t2.*2.85507460005156e+18;
t22 = -t20;
t23 = -t21;
t71 = -t55;
t78 = -t60;
t81 = -t62;
t83 = -t63;
t85 = -t66;
t89 = -t70;
t90 = -t73;
t95 = -t76;
t97 = -t79;
t100 = t8+t11+t14;
t101 = -t86;
t102 = -t87;
t106 = -t92;
t107 = -t96;
t108 = t9+t10+t15;
t109 = -t103;
t117 = t30+t36+t37+t40+t46+t47+1.42753730002578e+14;
t118 = t33+t35+t38+t44+t49+t53+7.1376865001289e+13;
t111 = t16+t19+t22-2.275477497e+9;
t112 = t17+t18+t23+3.0399800799e+10;
t119 = 1.0./t118;
t120 = 1.0./t117;
t113 = t111.^2;
t114 = t112.^2;
t115 = t100.*t111;
t116 = t108.*t112;
t121 = t110+t113+t114-2.569567140046404e+21;
t122 = t57+t115+t116;
t123 = t122.^2;
t125 = t118.*t121;
t124 = t123.*1.0e+4;
t126 = -t125;
t127 = t124+t126;
t128 = sqrt(t127);
t129 = t128./1.0e+2;
t130 = Z1.*t128.*3.799498679230342e-3;
t131 = Z1.*t128.*3.621952011976588e-2;
t132 = Z2.*t128.*1.535186849520796e-2;
t133 = Z3.*t128.*2.086765162455792e-2;
t134 = Z3.*t128.*3.049068098971141e-2;
t135 = Z2.*t128.*3.429017966894175e-2;
mt1 = [(t119.*(t61+t64+t65+t67+t72+t75+t77+t81+t82+t83+t84+t85+t90+t94+t98+t101+t105+t106+t130+t134-t135+1.922433295028705e+16))./2.0e+2,(t119.*(t61+t64+t65+t67+t72+t75+t77+t81+t82+t83+t84+t85+t90+t94+t98+t101+t105+t106-t130-t134+t135+1.922433295028705e+16))./2.0e+2,(t119.*(t54-t55+t56+t59-t60+t68+t69+t74+t89+t91+t93+t95+t97+t99+t102+t104+t107+t109+t131-t132-t133+3.556391874974202e+16))./2.0e+2];
mt2 = [(t119.*(t54+t56+t59+t68+t69+t71+t74+t78+t89+t91+t93+t95+t97+t99+t102+t104+t107+t109-t131+t132+t133+3.556391874974202e+16))./2.0e+2,t120.*(-t31-t32+t34+t39+t41-t42-t43+t45+t48+t50-t51-t52+t129)+3.0e+1,-t120.*(t31+t32-t34-t39-t41+t42+t43-t45-t48-t50+t51+t52+t129)+3.0e+1];
pv = reshape([mt1,mt2],2,3);

if pv(1,3)>0
    h=pv(1,3);
else
    h=pv(2,3);
end

== matlab function observe_2021a/trans_sensor_value2/MATLAB Function1 ==
  data: u input; y output
function y = fcn(u)
%u:光学センサの出力(V)、y:光学センサの出力PV値(mm)
    %出力スケーリングを行っています(フリーレンジ)。（光学センサの設定10,P.4-27）
    %PV値範囲を0～-50、出力電圧範囲を-5～5としているので、以下の式に従って
    %電圧値が距離に変換されます。
    y=(u-5*ones(3,1))*(-5);
% y = u;

== matlab function observe_2021a/MATLAB Function ==
  data: u input; y output
function y = fcn(u)
%u:光学センサの出力(V)、y:光学センサの出力PV値(mm)
    %出力スケーリングを行っています(フリーレンジ)。（光学センサの設定10,P.4-27）
    %PV値範囲を0～-50、出力電圧範囲を-5～5としているので、以下の式に従って
    %電圧値が距離に変換されます。
    y=(u-5*ones(3,1))*(-5);
% y = u;

== matlab function observe_2021a/trans_sensor_value2/autogen_Z2p1 ==
  data: Z1 input; h output; Z2 input; Z3 input
function h = autogen_Z2p(Z1,Z2,Z3)
%#codegen

%    This function was generated by the Symbolic Math Toolbox version 8.7.
%    09-Feb-2022 18:15:15

t2 = Z1.^2;
t3 = Z1.^3;
t4 = Z2.^2;
t5 = Z2.^3;
t6 = Z3.^2;
t7 = Z3.^3;
t8 = Z1.*3.21e+2;
t9 = Z2.*1.297e+3;
t10 = Z3.*1.763e+3;
t11 = Z3.*2.576e+3;
t12 = Z2.*2.897e+3;
t13 = Z1.*3.06e+3;
t24 = Z2.*Z3.*1.0352122e+11;
t25 = Z2.*Z3.*2.0704244e+11;
t26 = Z1.*Z3.*9.135768e+10;
t27 = Z1.*Z3.*1.8271536e+11;
t28 = Z1.*Z2.*1.9595028e+11;
t29 = Z1.*Z2.*9.797514e+10;
t39 = Z1.*4.8999911281101e+13;
t41 = Z3.*4.7733218776365e+13;
t48 = Z2.*4.6020599945112e+13;
t56 = Z1.*Z3.*2.511664935e+13;
t57 = Z1.*1.42753730002578e+14;
t58 = Z2.*Z3.*5.124007469e+13;
t68 = Z1.*Z2.*4.264372839e+13;
t80 = Z1.*Z2.*1.7692425141e+14;
t82 = Z1.*Z3.*1.4293441815e+14;
t88 = Z2.*Z3.*2.2089361633e+14;
t14 = -t12;
t15 = -t13;
t16 = t2.*3.21e+6;
t17 = t4.*1.297e+7;
t18 = t6.*1.763e+7;
t19 = t6.*2.576e+7;
t20 = t4.*2.897e+7;
t21 = t2.*3.06e+7;
t30 = t4.*2.0149636e+11;
t31 = Z1.*t6.*4.567884e+10;
t32 = Z3.*t2.*4.567884e+10;
t33 = t2.*9.466641e+10;
t34 = t3.*9.466641e+10;
t35 = -t24;
t36 = t2.*1.8933282e+11;
t37 = -t25;
t38 = -t26;
t40 = t6.*1.948789e+11;
t42 = Z2.*t6.*5.176061e+10;
t43 = Z3.*t4.*5.176061e+10;
t44 = t4.*1.0074818e+11;
t45 = t5.*1.0074818e+11;
t46 = -t27;
t47 = -t28;
t49 = t6.*9.743945e+10;
t50 = t7.*9.743945e+10;
t51 = Z1.*t4.*4.898757e+10;
t52 = Z2.*t2.*4.898757e+10;
t53 = -t29;
t54 = Z2.*t3.*3.21e+10;
t55 = Z3.*t3.*3.21e+10;
t59 = Z1.*t7.*2.576e+11;
t60 = Z2.*t7.*2.576e+11;
t61 = Z1.*t7.*1.763e+11;
t62 = Z2.*t7.*1.763e+11;
t63 = Z1.*t5.*1.297e+11;
t64 = Z3.*t5.*1.297e+11;
t65 = Z2.*Z3.*t2.*4.66e+10;
t66 = Z2.*t3.*3.06e+11;
t67 = Z3.*t3.*3.06e+11;
t69 = Z1.*t5.*2.897e+11;
t70 = Z3.*t5.*2.897e+11;
t72 = t2.*1.699491663e+13;
t73 = Z1.*Z3.*t4.*4.823e+11;
t74 = Z2.*Z3.*t2.*5.473e+11;
t75 = Z1.*Z2.*t6.*4.357e+11;
t76 = Z1.*Z3.*t4.*2.255e+11;
t77 = -t58;
t79 = t2.*3.388018887e+13;
t84 = t4.*t6.*4.66e+10;
t86 = t6.*4.584717173e+13;
t87 = Z1.*Z2.*t6.*3.218e+11;
t91 = t4.*8.912494397e+13;
t92 = t2.*t6.*4.823e+11;
t93 = t4.*t6.*5.473e+11;
t94 = t2.*t4.*4.357e+11;
t96 = t2.*t6.*2.255e+11;
t98 = -t80;
t99 = t6.*9.788848349e+13;
t103 = t2.*t4.*3.218e+11;
t104 = -t88;
t105 = t4.*1.1408216305e+14;
t110 = t2.*2.85507460005156e+18;
t22 = -t20;
t23 = -t21;
t71 = -t55;
t78 = -t60;
t81 = -t62;
t83 = -t63;
t85 = -t66;
t89 = -t70;
t90 = -t73;
t95 = -t76;
t97 = -t79;
t100 = t8+t11+t14;
t101 = -t86;
t102 = -t87;
t106 = -t92;
t107 = -t96;
t108 = t9+t10+t15;
t109 = -t103;
t117 = t30+t36+t37+t40+t46+t47+1.42753730002578e+14;
t118 = t33+t35+t38+t44+t49+t53+7.1376865001289e+13;
t111 = t16+t19+t22-2.275477497e+9;
t112 = t17+t18+t23+3.0399800799e+10;
t119 = 1.0./t118;
t120 = 1.0./t117;
t113 = t111.^2;
t114 = t112.^2;
t115 = t100.*t111;
t116 = t108.*t112;
t121 = t110+t113+t114-2.569567140046404e+21;
t122 = t57+t115+t116;
t123 = t122.^2;
t125 = t118.*t121;
t124 = t123.*1.0e+4;
t126 = -t125;
t127 = t124+t126;
t128 = sqrt(t127);
t129 = t128./1.0e+2;
t130 = Z1.*t128.*3.799498679230342e-3;
t131 = Z1.*t128.*3.621952011976588e-2;
t132 = Z2.*t128.*1.535186849520796e-2;
t133 = Z3.*t128.*2.086765162455792e-2;
t134 = Z3.*t128.*3.049068098971141e-2;
t135 = Z2.*t128.*3.429017966894175e-2;
mt1 = [(t119.*(t61+t64+t65+t67+t72+t75+t77+t81+t82+t83+t84+t85+t90+t94+t98+t101+t105+t106+t130+t134-t135+1.922433295028705e+16))./2.0e+2,(t119.*(t61+t64+t65+t67+t72+t75+t77+t81+t82+t83+t84+t85+t90+t94+t98+t101+t105+t106-t130-t134+t135+1.922433295028705e+16))./2.0e+2,(t119.*(t54-t55+t56+t59-t60+t68+t69+t74+t89+t91+t93+t95+t97+t99+t102+t104+t107+t109+t131-t132-t133+3.556391874974202e+16))./2.0e+2];
mt2 = [(t119.*(t54+t56+t59+t68+t69+t71+t74+t78+t89+t91+t93+t95+t97+t99+t102+t104+t107+t109-t131+t132+t133+3.556391874974202e+16))./2.0e+2,t120.*(-t31-t32+t34+t39+t41-t42-t43+t45+t48+t50-t51-t52+t129)+3.0e+1,-t120.*(t31+t32-t34-t39-t41+t42+t43-t45-t48-t50+t51+t52+t129)+3.0e+1];
pv = reshape([mt1,mt2],2,3);

if pv(1,3)>0
    h=pv(1,3);
else
    h=pv(2,3);
end
